simulink model "schema di desaturazione dell_azione di comando"  (R2016a)
settings: Solver=ode3  StartTime=0.0  StopTime=200  FixedStep=0.1  RelTol=1e-5
libraries: simulink x3
settings Model: Creator=The MathWorks, Inc.  LastModifiedBy=User
settings SolverCC: MaxConsecutiveZCs=100000  ZeroCrossAlgorithm=Adaptive
settings DataIOCC: LimitDataPoints=on  MaxDataPoints=100000  SaveFormat=Array
settings OptimizationCC: ExpressionDepthLimit=2147483647
settings DebuggingCC: UnderspecifiedInitializationDetection=Classic  MergeDetectMultiDrivingBlocksExec=none  FcnCallInpInsideContextMsg=UseLocalSettings  StateNameClashWarn=warning
settings HardwareCC: ProdBitPerPointer=32  ProdLargestAtomicFloat=None  ProdIntDivRoundTo=Undefined  ProdEndianess=Unspecified  ProdWordSize=32  ProdHWDeviceType=32-bit Generic
settings ModelReferenceCC: PropagateSignalLabelsOutOfModel=off
settings GRTTargetCC: CombineOutputUpdateFcns=off  GRTInterface=on
settings ConfigComp: CovModelRefEnable=Off

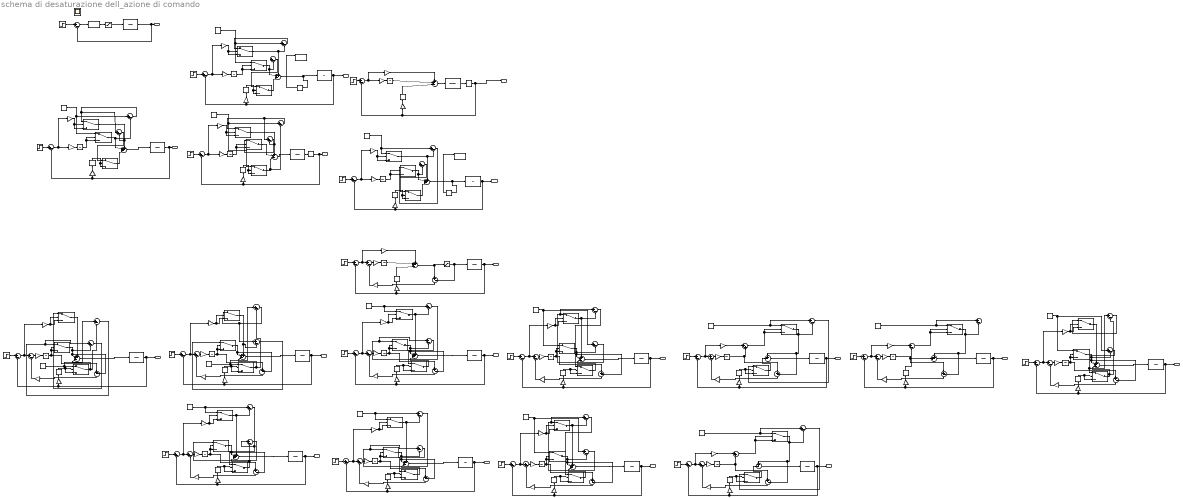
== system schema di desaturazione dell_azione di comando ==
  note: DESATURAZIONE CLASSICA
  note: TASK P, poi I,poi D
  note: TASK I,poi P,poi D
  note: PI
  note: Anti-Windup PID Control Demonstration
  note: TASK P(alternativo)
  note: TASK I(alternativo)
  note: PI(alternativo)
  note: TASK D, poi P,poi I
  note: TASK P, poi D, poi I
  note: TASK I,poi D,poi P
  note: TASK D, poi I,poi P
  note: PD
  Constant{,2..3,5..11,13..15} (13 alike) : Constant  Value=1.05
  Constant1 : Constant  Value=1.5
  Constant4 : Constant  Value=10
  DERIVATIVE{1..14,16..18} (17 alike) : Derivative
  Dead Time : TransportDelay  BufferSize=2048
  Dead Time1 : TransportDelay  BufferSize=2048
  First Order Process{,1,4,6..9,13..14,16..18} (12 alike) : TransferFcn  Numerator=1  Denominator=[1 0 0]
  First Order Process10 : TransferFcn  Numerator=1  Denominator=[1 0]
  First Order Process11 : TransferFcn  Numerator=1  Denominator=[1 1]
  First Order Process12 : TransferFcn  Numerator=1  Denominator=[1 1]
  First Order Process2 : TransferFcn  Numerator=1  Denominator=[1 1 0]
  First Order Process3 : TransferFcn  Numerator=1  Denominator=[1 0]
  First Order Process5 : TransferFcn  Numerator=1  Denominator=[1 0]
  INTEGRATOR{1..14,16..18} (17 alike) : Integrator
  Kd{1,4,10..12} (5 alike) : Gain  Gain=0
  Kd{5..9,13..14,16..18} (10 alike) : Gain  Gain=10
  Kd2 : Gain  Gain=0.9
  Kd3 : Gain  Gain=0.9
  Ki{1,4..10,13..14,16..18} (13 alike) : Gain  Gain=10
  Ki11 : Gain  Gain=2
  Ki12 : Gain  Gain=2
  Ki2 : Gain  Gain=0.036
  Ki3 : Gain  Gain=0.036
  Kp{1,4..9,13..14,16..18} (12 alike) : Gain  Gain=10
  Kp10 : Gain  Gain=2
  Kp11 : Gain  Gain=2
  Kp12 : Gain  Gain=2
  Kp2 : Gain  Gain=0.37
  Kp3 : Gain  Gain=0.37
  Memory : Memory
  Memory1 : Memory
  MinMax Running Resettable : simulink/Math Operations/MinMax Running Resettable  Function=max  vinit=0.0
  MinMax Running Resettable1 : simulink/Math Operations/MinMax Running Resettable  Function=max  vinit=0.0
  PID Controller : simulink/Continuous/PID Controller  Controller=PID  TimeDomain=Continuous-time  SampleTime=-1  IntegratorMethod=Forward Euler  FilterMethod=Forward Euler  Form=Parallel  UseFilter=on  ControllerParametersSource=internal  P=10  I=10  D=10  N=5  InitialConditionSource=internal  InitialConditionForIntegrator=0  InitialConditionForFilter=0  ExternalReset=none  LimitOutput=off  UpperSaturationLimit=10  LowerSaturationLimit=-10  LinearizeAsGain=off  AntiWindupMode=none  Kb=1  TrackingMode=off  Kt=1  PParamMin=[]  PParamMax=[]  IParamMin=[]  IParamMax=[]  DParamMin=[]  DParamMax=[]  NParamMin=[]  NParamMax=[]  KbParamMin=[]  KbParamMax=[]  KtParamMin=[]  KtParamMax=[]  POutMin=[]  POutMax=[]  IOutMin=[]  IOutMax=[]  DOutMin=[]  DOutMax=[]  NOutMin=[]  NOutMax=[]  KbOutMin=[]  KbOutMax=[]  KtOutMin=[]  KtOutMax=[]  IntegratorOutMin=[]  IntegratorOutMax=[]  FilterOutMin=[]  FilterOutMax=[]  SumOutMin=[]  SumOutMax=[]  SumI1OutMin=[]  SumI1OutMax=[]  SumI2OutMin=[]  SumI2OutMax=[]  SumI3OutMin=[]  SumI3OutMax=[]  SumDOutMin=[]  SumDOutMax=[]  SaturationOutMin=[]  SaturationOutMax=[]  IntegratorContinuousStateAttributes=''  IntegratorStateMustResolveToSignalObject=off  IntegratorRTWStateStorageClass=Auto  FilterContinuousStateAttributes=''  FilterStateMustResolveToSignalObject=off  FilterRTWStateStorageClass=Auto  DifferentiatorICPrevScaledInput=0  DifferentiatorOutMin=[]  DifferentiatorOutMax=[]
  Saturation : Saturate  UpperLimit=1.05  LowerLimit=-1.05
  Saturation1 : Saturate  UpperLimit=1.05  LowerLimit=-1.05
  Step{,1..14,16..18} (18 alike) : Step  SampleTime=0
  Sum{,1..4,6..8,10..11,13..15,17,19..21,23..27,29..31,33..37,39,41..43,45..49,51..55,57,59..61,63..67,69..70,77..79,81..85,87..91,93..94} (70 alike) : Sum  Inputs=|+-
  Sum{5,9,12,16,18,22,28,32,44,50,62,68,80,86} (14 alike) : Sum  Inputs=++-|
  Sum38 : Sum  Inputs=+-|
  Sum40 : Sum  Inputs=|++
  Sum56 : Sum  Inputs=+-|
  Sum58 : Sum  Inputs=|++
  Sum92 : Sum  Inputs=++|
  Switch{,1..2,6..11,15..33,36..41,43} (35 alike) : Switch  Threshold=1.05
  Switch12 : Switch  Threshold=10
  Switch13 : Switch  Threshold=10
  Switch14 : Switch  Threshold=10
  Switch3 : Switch  Threshold=1.5
  Switch4 : Switch  Threshold=1.5
  Switch5 : Switch  Threshold=1.5
  ka{,1..8,10..12} (12 alike) : Gain
  yout : Outport
  yout5 : Outport  Port=2
  yout2 : Outport  Port=3
  yout6 : Outport  Port=4
  yout1 : Outport  Port=5
  yout3 : Outport  Port=6
  yout4 : Outport  Port=7
  yout7 : Outport  Port=8
  yout8 : Outport  Port=9
  yout9 : Outport  Port=10
  yout10 : Outport  Port=11
  yout11 : Outport  Port=12
  yout12 : Outport  Port=13
  yout13 : Outport  Port=14
  yout14 : Outport  Port=15
  yout16 : Outport  Port=16
  yout17 : Outport  Port=17
  yout18 : Outport  Port=18
  Scope : Scope
  Scope1 : Scope
  wires:
  Step/1 -> Sum/1  "r(t)"
  Sum/1 -> PID Controller/1  "e(t)"
  First Order Process/1 -> yout/1, Sum/2  "y(t)"
  Step5/1 -> Sum10/1  "r(t)"
  Sum10/1 -> Ki1/1, Kp1/1  "e(t)"
  First Order Process5/1 -> yout5/1, Kd1/1, Sum10/2  "yintegrat(t)"
  Ki1/1 -> INTEGRATOR1/1
  Kd1/1 -> DERIVATIVE1/1
  Kp1/1 -> Switch/3, Switch/2
  Switch/1 -> Sum1/2, Sum12/1
  Switch2/1 -> Sum12/3
  DERIVATIVE1/1 -> Switch2/2, Switch2/3
  INTEGRATOR1/1 -> Switch1/3, Switch1/2  "u(t)"
  Switch1/1 -> Sum2/2, Sum12/2
  Sum2/1 -> Switch2/1
  Step2/1 -> Sum14/1  "r(t)"
  Sum14/1 -> Ki3/1, Kp3/1  "e(t)"
  Ki3/1 -> INTEGRATOR3/1
  Kd3/1 -> DERIVATIVE3/1
  INTEGRATOR3/1 -> Sum16/2  "u(t)"
  Kp3/1 -> Sum16/1
  DERIVATIVE3/1 -> Sum16/3
  PID Controller/1 -> Saturation/1  "u(t)"
  Saturation/1 -> First Order Process/1
  Sum12/1 -> Memory/1, First Order Process5/1  "u(t)"
  Step6/1 -> Sum26/1  "r(t)"
  Sum26/1 -> Ki6/1, Kp6/1  "e(t)"
  First Order Process6/1 -> yout6/1, Kd6/1, Sum26/2  "yint(t)"
  Ki6/1 -> INTEGRATOR6/1
  Kd6/1 -> DERIVATIVE6/1
  Constant4/1 -> Switch13/1, Sum25/1
  Kp6/1 -> Switch12/3, Switch12/2
  Switch14/1 -> Sum28/3
  DERIVATIVE6/1 -> Switch14/2, Switch14/3
  INTEGRATOR6/1 -> Switch13/3, Switch13/2  "u(t)"
  Sum30/1 -> Switch14/1
  Sum25/1 -> Sum30/1, Switch12/1
  Switch13/1 -> Sum25/2, Sum28/2
  Switch12/1 -> Sum30/2, Sum28/1
  Sum28/1 -> First Order Process6/1  "u(t)"
  Step1/1 -> Sum4/1  "r(t)"
  Sum4/1 -> Ki2/1, Kp2/1  "e(t)"
  First Order Process1/1 -> Dead Time1/1  "yder(t)"
  Ki2/1 -> INTEGRATOR2/1
  Kd2/1 -> DERIVATIVE2/1
  Kp2/1 -> Switch3/3, Switch3/2
  Switch5/1 -> Sum3/2, Sum5/3
  DERIVATIVE2/1 -> Switch5/2, Switch5/3
  INTEGRATOR2/1 -> Switch4/3, Switch4/2  "u(t)"
  Switch4/1 -> Sum5/2
  Switch3/1 -> Sum6/2, Sum5/1
  Sum5/1 -> First Order Process1/1  "u(t)"
  Constant1/1 -> Sum3/1, Switch5/1
  Sum3/1 -> Switch3/1, Sum6/1
  Sum6/1 -> Switch4/1
  Sum16/1 -> First Order Process2/1  "u(t)"
  First Order Process2/1 -> Dead Time/1  "yrit(t)"
  Dead Time/1 -> yout2/1, Kd3/1, Sum14/2
  Dead Time1/1 -> yout1/1, Kd2/1, Sum4/2
  Memory/1 -> MinMax Running Resettable/1
  Sum1/1 -> Switch/1
  Constant/1 -> Sum1/1, Switch1/1
  Step3/1 -> Sum8/1  "r(t)"
  Sum8/1 -> Ki4/1, Kp4/1  "e(t)"
  First Order Process3/1 -> yout3/1, Kd4/1, Sum8/2  "yprop(t)"
  Ki4/1 -> INTEGRATOR4/1
  Kd4/1 -> DERIVATIVE4/1
  Kp4/1 -> Switch6/3, Switch6/2
  Switch6/1 -> Sum7/2, Sum9/1
  Switch8/1 -> Sum9/3
  DERIVATIVE4/1 -> Switch8/2, Switch8/3
  INTEGRATOR4/1 -> Switch7/3, Switch7/2  "u(t)"
  Switch7/1 -> Sum11/2, Sum9/2
  Sum11/1 -> Switch8/1
  Sum9/1 -> Memory1/1, First Order Process3/1  "u(t)"
  Memory1/1 -> MinMax Running Resettable1/1
  Constant2/1 -> Sum7/1, Switch6/1
  Sum7/1 -> Switch7/1
  Step4/1 -> Sum17/1  "r(t)"
  Sum17/1 -> Sum13/1, Kp5/1  "e(t)"
  First Order Process4/1 -> yout4/1, Kd5/1, Sum17/2  "ydesat(t)"
  Ki5/1 -> INTEGRATOR5/1
  Kd5/1 -> DERIVATIVE5/1
  Sum18/1 -> Sum15/1, Saturation1/1  "u(t)"
  Sum13/1 -> Ki5/1
  Saturation1/1 -> Sum15/2, First Order Process4/1
  Sum15/1 -> ka/1
  DERIVATIVE5/1 -> Sum18/3
  INTEGRATOR5/1 -> Sum18/2  "u(t)"
  Kp5/1 -> Sum18/1
  ka/1 -> Sum13/2
  Step7/1 -> Sum21/1  "r(t)"
  Sum21/1 -> Sum19/1, Kp7/1  "e(t)"
  First Order Process7/1 -> yout7/1, Kd7/1, Sum21/2  "ydesat_taskP, poi I, poi D(t)"
  Ki7/1 -> INTEGRATOR7/1
  Kd7/1 -> DERIVATIVE7/1
  Sum22/1 -> First Order Process7/1  "u(t)"
  Sum19/1 -> Ki7/1
  Sum20/1 -> ka1/1
  INTEGRATOR7/1 -> Sum20/1, Switch10/3, Switch10/2  "u(t)"
  Kp7/1 -> Switch9/2, Switch9/3
  ka1/1 -> Sum19/2
  Constant3/1 -> Sum23/1, Switch9/1
  Switch9/1 -> Sum23/2, Sum22/1
  Sum23/1 -> Sum24/1, Switch10/1
  Switch10/1 -> Sum24/2, Sum22/2, Sum20/2
  DERIVATIVE7/1 -> Switch11/2, Switch11/3
  Sum24/1 -> Switch11/1
  Switch11/1 -> Sum22/3
  Step8/1 -> Sum31/1  "r(t)"
  Sum31/1 -> Sum27/1, Kp8/1  "e(t)"
  First Order Process8/1 -> yout8/1, Kd8/1, Sum31/2  "ydesat_task_I,poi P,poi D(t)"
  Ki8/1 -> INTEGRATOR8/1
  Kd8/1 -> DERIVATIVE8/1
  Sum32/1 -> First Order Process8/1  "u(t)"
  Sum27/1 -> Ki8/1
  Sum29/1 -> ka2/1
  INTEGRATOR8/1 -> Sum29/1, Switch15/3, Switch15/2  "u(t)"
  Kp8/1 -> Switch17/2, Switch17/3
  ka2/1 -> Sum27/2
  Switch17/1 -> Sum33/2, Sum32/1
  DERIVATIVE8/1 -> Switch16/2, Switch16/3
  Switch16/1 -> Sum32/3
  Constant5/1 -> Sum34/1, Switch15/1
  Sum34/1 -> Sum33/1, Switch17/1
  Sum33/1 -> Switch16/1
  Step9/1 -> Sum37/1  "r(t)"
  Sum37/1 -> Sum35/1, Kp9/1  "e(t)"
  First Order Process9/1 -> yout9/1, Kd9/1, Sum37/2  "y(t)desatPI"
  Ki9/1 -> INTEGRATOR9/1
  Kd9/1 -> DERIVATIVE9/1
  Sum35/1 -> Ki9/1
  Sum36/1 -> ka3/1
  ka3/1 -> Sum35/2
  DERIVATIVE9/1 -> Switch19/2, Switch19/3
  Switch19/1 -> Sum38/2
  INTEGRATOR9/1 -> Sum36/1, Sum40/2  "u(t)"
  Kp9/1 -> Sum40/1
  Sum40/1 -> Switch20/3, Switch20/2
  Constant6/1 -> Sum39/1, Switch20/1
  Switch20/1 -> Sum39/2, Sum36/2, Sum38/1
  Sum39/1 -> Switch19/1
  Switch15/1 -> Sum34/2, Sum29/2, Sum32/2
  Sum38/1 -> First Order Process9/1  "u(t)"
  Step10/1 -> Sum43/1  "r(t)"
  Sum43/1 -> Sum41/1, Kp10/1  "e(t)"
  First Order Process10/1 -> yout10/1, Kd10/1, Sum43/2  "ydesat_taskP(alternativo)(t)"
  Ki10/1 -> INTEGRATOR10/1
  Kd10/1 -> DERIVATIVE10/1
  Sum44/1 -> First Order Process10/1  "u(t)"
  Sum41/1 -> Ki10/1
  Sum42/1 -> ka4/1
  INTEGRATOR10/1 -> Sum42/1, Switch18/3, Switch18/2  "u(t)"
  Kp10/1 -> Switch27/2, Switch27/3
  ka4/1 -> Sum41/2
  Constant7/1 -> Sum45/1, Switch27/1
  Switch27/1 -> Sum45/2, Sum44/1
  Sum45/1 -> Sum46/1, Switch18/1
  Switch18/1 -> Sum46/2, Sum44/2, Sum42/2
  DERIVATIVE10/1 -> Switch21/2, Switch21/3
  Sum46/1 -> Switch21/1
  Switch21/1 -> Sum44/3
  Step11/1 -> Sum49/1  "r(t)"
  Sum49/1 -> Sum47/1, Kp11/1  "e(t)"
  First Order Process11/1 -> yout11/1, Kd11/1, Sum49/2  "ydesat_task_I(alternativo)(t)"
  Ki11/1 -> INTEGRATOR11/1
  Kd11/1 -> DERIVATIVE11/1
  Sum50/1 -> First Order Process11/1  "u(t)"
  Sum47/1 -> Ki11/1
  Sum48/1 -> ka5/1
  INTEGRATOR11/1 -> Sum48/1, Switch22/3, Switch22/2  "u(t)"
  Kp11/1 -> Switch24/2, Switch24/3
  ka5/1 -> Sum47/2
  Switch24/1 -> Sum51/2, Sum50/1
  DERIVATIVE11/1 -> Switch23/2, Switch23/3
  Switch23/1 -> Sum50/3
  Constant8/1 -> Sum52/1, Switch22/1
  Sum52/1 -> Sum51/1, Switch24/1
  Sum51/1 -> Switch23/1
  Step12/1 -> Sum55/1  "r(t)"
  Sum55/1 -> Sum53/1, Kp12/1  "e(t)"
  First Order Process12/1 -> yout12/1, Kd12/1, Sum55/2  "ydesat_taskPI(alternativo)(t)"
  Ki12/1 -> INTEGRATOR12/1
  Kd12/1 -> DERIVATIVE12/1
  Sum53/1 -> Ki12/1
  Sum54/1 -> ka6/1
  ka6/1 -> Sum53/2
  DERIVATIVE12/1 -> Switch25/2, Switch25/3
  Switch25/1 -> Sum56/2
  INTEGRATOR12/1 -> Sum54/1, Sum58/2  "u(t)"
  Kp12/1 -> Sum58/1
  Sum58/1 -> Switch26/3, Switch26/2
  Constant9/1 -> Sum57/1, Switch26/1
  Switch26/1 -> Sum57/2, Sum54/2, Sum56/1
  Sum57/1 -> Switch25/1
  Switch22/1 -> Sum52/2, Sum48/2, Sum50/2
  Sum56/1 -> First Order Process12/1  "u(t)"
  Step13/1 -> Sum61/1  "r(t)"
  Sum61/1 -> Sum59/1, Kp13/1  "e(t)"
  First Order Process13/1 -> yout13/1, Kd13/1, Sum61/2  "ydesat_taskD,poi P,poi I(t)"
  Ki13/1 -> INTEGRATOR13/1
  Kd13/1 -> DERIVATIVE13/1
  Sum62/1 -> First Order Process13/1  "u(t)"
  Sum59/1 -> Ki13/1
  Sum60/1 -> ka7/1
  INTEGRATOR13/1 -> Sum60/1, Switch28/3, Switch28/2  "u(t)"
  Kp13/1 -> Switch30/2, Switch30/3
  ka7/1 -> Sum59/2
  Switch30/1 -> Sum64/2, Sum62/1
  Switch28/1 -> Sum62/2, Sum60/2
  DERIVATIVE13/1 -> Switch29/2, Switch29/3
  Switch29/1 -> Sum63/2, Sum62/3
  Constant10/1 -> Sum63/1, Switch29/1
  Sum63/1 -> Switch30/1, Sum64/1
  Sum64/1 -> Switch28/1
  Step14/1 -> Sum67/1  "r(t)"
  Sum67/1 -> Sum65/1, Kp14/1  "e(t)"
  First Order Process14/1 -> yout14/1, Kd14/1, Sum67/2  "ydesat_taskP poi D poi I(t)"
  Ki14/1 -> INTEGRATOR14/1
  Kd14/1 -> DERIVATIVE14/1
  Sum68/1 -> First Order Process14/1  "u(t)"
  Sum65/1 -> Ki14/1
  Sum66/1 -> ka8/1
  INTEGRATOR14/1 -> Sum66/1, Switch31/3, Switch31/2  "u(t)"
  Kp14/1 -> Switch33/2, Switch33/3
  ka8/1 -> Sum65/2
  Constant11/1 -> Sum69/1, Switch33/1
  Switch33/1 -> Sum69/2, Sum68/1
  Switch31/1 -> Sum68/2, Sum66/2
  DERIVATIVE14/1 -> Switch32/2, Switch32/3
  Switch32/1 -> Sum68/3, Sum70/2
  Sum69/1 -> Sum70/1, Switch32/1
  Sum70/1 -> Switch31/1
  Step16/1 -> Sum79/1  "r(t)"
  Sum79/1 -> Sum77/1, Kp16/1  "e(t)"
  First Order Process16/1 -> yout16/1, Kd16/1, Sum79/2  "ydesat_task_I,poi D,poi P(t)"
  Ki16/1 -> INTEGRATOR16/1
  Kd16/1 -> DERIVATIVE16/1
  Sum80/1 -> First Order Process16/1  "u(t)"
  Sum77/1 -> Ki16/1
  Sum78/1 -> ka10/1
  INTEGRATOR16/1 -> Sum78/1, Switch36/3, Switch36/2  "u(t)"
  Kp16/1 -> Switch38/2, Switch38/3
  ka10/1 -> Sum77/2
  Switch38/1 -> Sum80/1
  DERIVATIVE16/1 -> Switch37/2, Switch37/3
  Switch37/1 -> Sum81/2, Sum80/3
  Constant13/1 -> Sum82/1, Switch36/1
  Switch36/1 -> Sum82/2, Sum78/2, Sum80/2
  Sum82/1 -> Switch37/1, Sum81/1
  Sum81/1 -> Switch38/1
  Step17/1 -> Sum85/1  "r(t)"
  Sum85/1 -> Sum83/1, Kp17/1  "e(t)"
  First Order Process17/1 -> yout17/1, Kd17/1, Sum85/2  "ydesat_taskD,poi I,poi P(t)"
  Ki17/1 -> INTEGRATOR17/1
  Kd17/1 -> DERIVATIVE17/1
  Sum86/1 -> First Order Process17/1  "u(t)"
  Sum83/1 -> Ki17/1
  Sum84/1 -> ka11/1
  INTEGRATOR17/1 -> Sum84/1, Switch39/3, Switch39/2  "u(t)"
  Kp17/1 -> Switch41/2, Switch41/3
  ka11/1 -> Sum83/2
  Switch41/1 -> Sum86/1
  Switch39/1 -> Sum88/2, Sum86/2, Sum84/2
  DERIVATIVE17/1 -> Switch40/2, Switch40/3
  Switch40/1 -> Sum87/2, Sum86/3
  Constant14/1 -> Sum87/1, Switch40/1
  Sum87/1 -> Sum88/1, Switch39/1
  Sum88/1 -> Switch41/1
  Step18/1 -> Sum91/1  "r(t)"
  Sum91/1 -> Sum89/1, Kp18/1  "e(t)"
  First Order Process18/1 -> yout18/1, Kd18/1, Sum91/2  "y(t)desatPD SENZA I"
  Ki18/1 -> INTEGRATOR18/1
  Kd18/1 -> DERIVATIVE18/1
  Sum89/1 -> Ki18/1
  Sum90/1 -> ka12/1
  ka12/1 -> Sum89/2
  INTEGRATOR18/1 -> Sum92/2, Sum90/1  "u(t)"
  Kp18/1 -> Sum94/1
  Sum94/1 -> Switch43/3, Switch43/2
  Constant15/1 -> Sum93/1, Switch43/1
  Switch43/1 -> Sum93/2, Sum90/2, Sum92/1
  Sum92/1 -> First Order Process18/1  "u(t)"
  DERIVATIVE18/1 -> Sum94/2
